simulink model "GunnerusDP_v1"  (R2017b)
settings: Solver=ode4  StartTime=0.0  StopTime=Tsim  FixedStep=ts  RelTol=1e-3  EnableMultiTasking=on
values from neighbouring files (symbols this model uses):
  ts = 0.01    [InitGunnerusDP.m]
undefined symbols (not defined in the file or in its folder): Control, Current, Hoerner, Par, Sim, TC_currentChange, vessel, vesselABC
libraries: marine_hydro x4, marine_gnc x3, simulink x3
(part 1 of 4)
settings Model: Creator=Thor  LastModifiedBy=astrbro
settings DataIOCC: LimitDataPoints=on  SaveFormat=Array  SignalLoggingSaveFormat=ModelDataLogs
settings OptimizationCC: ExpressionDepthLimit=2147483647  InitFltsAndDblsToZero=on  LifeSpan=inf
settings DebuggingCC: SaveWithParameterizedLinksMsg=none  UnderspecifiedInitializationDetection=Classic  MergeDetectMultiDrivingBlocksExec=none  SignalResolutionControl=TryResolveAllWithWarning  SolverPrmCheckMsg=warning  MultiTaskDSMMsg=warning  MultiTaskCondExecSysMsg=none  MultiTaskRateTransMsg=warning  FcnCallInpInsideContextMsg=warning  StateNameClashWarn=warning  SFUnexpectedBacktrackingDiag=warning  SFNoUnconditionalDefaultTransitionDiag=warning  SFExecutionAtInitializationDiag=none
settings HardwareCC: ProdBitPerPointer=32  ProdBitPerSizeT=32  ProdBitPerPtrDiffT=32  ProdLargestAtomicFloat=None  ProdIntDivRoundTo=Undefined  ProdEndianess=Unspecified  ProdWordSize=32  ProdHWDeviceType=32-bit Generic
settings ModelReferenceCC: PropagateSignalLabelsOutOfModel=off
settings CodeAppCC: StateflowObjectComments=on
settings GRTTargetCC: TargetFcnLib=ansi_tfl_tmw.mat  TargetLangStandard=C89/C90 (ANSI)  GeneratePreprocessorConditionals=Disable all  CombineOutputUpdateFcns=off  GRTInterface=on
settings ConfigComp: CovMetricSettings=dw  CovHtmlReporting=on  CovSaveCumulativeToWorkspaceVar=on  CovSaveSingleToWorkspaceVar=on  CovExternalEMLEnable=off  CovSFcnEnable=off

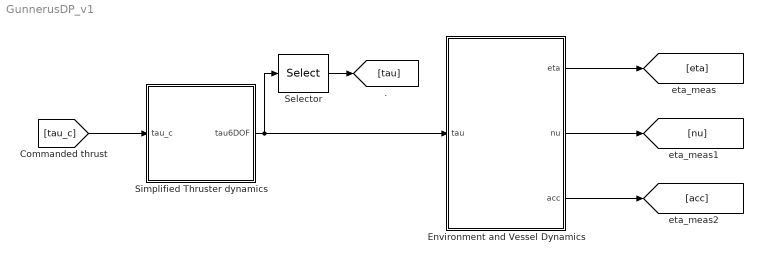
== system GunnerusDP_v1 ==
  Environment and Vessel Dynamics : Subsystem
  Selector : Selector  InputPortWidth=6  IndexOptions=Index vector (dialog)  Indices=[1 2 6]  OutputSizes=1
  Simplified Thruster dynamics : Subsystem
  wires:
  Selector/1 -> [tau]
  [tau_c] -> Simplified Thruster dynamics/1(tau_c)
  Simplified Thruster dynamics/1(tau6DOF) -> Selector/1, Environment and Vessel Dynamics/1(tau)
  Environment and Vessel Dynamics/2(nu) -> [nu]
  Environment and Vessel Dynamics/3(acc) -> [acc]
  Environment and Vessel Dynamics/1(eta) -> [eta]

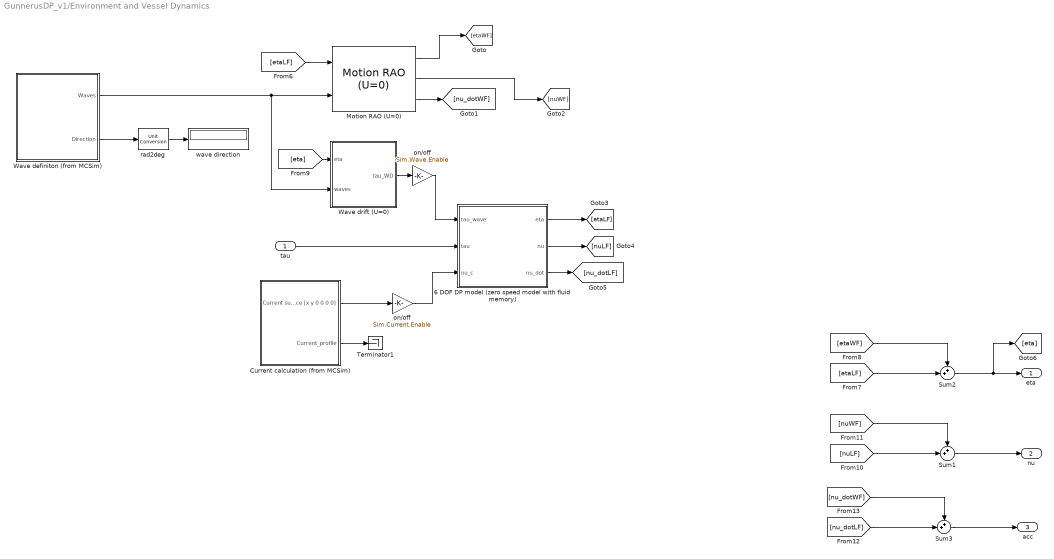
== system GunnerusDP_v1/Environment and Vessel Dynamics ==
  tau : Inport
  6 DOF DP model (zero speed model with fluid memory) : Subsystem  AncestorBlock=|  mask(6 DOF zero speed model){ABC=vesselABC, rho=1025, Axc=106, Ayc=419, CX=1.0, CY_2D=Hoerner(vessel.main.B,vessel.main.T), Bv=vessel.Bv, Dp=vesselABC.Dp}
      | marine_hydro/Hydro Library/6 DOF DP model
      |  (zero speed model with fluid memory)
      mask prompts: ABC "Structure containing model parameters and the fluid memory effects"; rho "Density of water (kg/m3)"; Axc "Frontal projected current area Axc (m2)"; Ayc "Laterall projected current area Ayc (m2)"; CX "Current (drag) coefficient in surge CX"; CY_2D "2D drag coefficient in sway CY_2D"; Bv "Linear viscous damping matrix"; Dp "Linear potential damping matrix"
      mask help: System block containing the zero speed 6 DOF equations of motion including fluid memory effetcs.
  Current calculation (from MCSim) : Subsystem
  Motion RAO (U=0) : marine_hydro/Hydro Library/Motion RAO (U=0)  RAO_Freq=vessel.motionRAO.w  RAO_Dir=vessel.headings  RAO_Vel=vessel.velocities  RAO_Amp=vessel.motionRAO.amp  RAO_Phase=vessel.motionRAO.phase  RAO_add_omega_0=on  RAO_add_omega_inf=on  RAO_yaw_quantization_flag=on  RAO_yaw_quant=5*pi/180  RAO_yaw_back=1.2*pi/180  RAO_speed_backlash_flag=on  RAO_speed_back=2  RAO_smoothing_flag=on
      settings: SourceProductName=MSS Hydro
  Sum1 : Sum  Inputs=++|
  Sum2 : Sum  Inputs=++|
  Sum3 : Sum  Inputs=++|
  Terminator1 : Terminator
  Wave definiton (from MCSim) : Subsystem
  Wave drift (U=0) : Subsystem  AncestorBlock=marine_hydro/Hydro Library/Wave drift (U=0)
  on/off : Gain  Gain=Sim.Wave.Enable
  "on/off " : Gain  Gain=Sim.Current.Enable
  rad2deg : marine_gnc/Utilities/Math Operations/Unit Conversion  in=rad2deg
      settings: SourceProductName=MSS GNC
  wave direction : Display
  eta : Outport
  nu : Outport  Port=2
  acc : Outport  Port=3
  wires:
  Current calculation (from MCSim)/2(Current_profile) -> Terminator1/1
  Wave drift (U=0)/1(tau_WD) -> on/off/1
  on/off/1 -> 6 DOF DP model (zero speed model with fluid memory)/1(tau_wave)
  "on/off "/1 -> 6 DOF DP model (zero speed model with fluid memory)/3(nu_c)
  Current calculation (from MCSim)/1(Current surface [x y 0 0 0 0]) -> "on/off "/1
  Motion RAO (U=0)/3 -> [nu_dotWF]
  Motion RAO (U=0)/2 -> [nuWF]
  Motion RAO (U=0)/1 -> [etaWF]
  rad2deg/1 -> wave direction/1
  Wave definiton (from MCSim)/2(Direction) -> rad2deg/1
  Wave definiton (from MCSim)/1(Waves) -> Motion RAO (U=0)/2, Wave drift (U=0)/2(waves)
  6 DOF DP model (zero speed model with fluid memory)/1(eta) -> [etaLF]
  tau/1 -> 6 DOF DP model (zero speed model with fluid memory)/2(tau)
  6 DOF DP model (zero speed model with fluid memory)/3(nu_dot) -> [nu_dotLF]
  6 DOF DP model (zero speed model with fluid memory)/2(nu) -> [nuLF]
  [etaLF] -> Motion RAO (U=0)/1
  [etaLF] -> Sum2/2
  [etaWF] -> Sum2/1
  Sum2/1 -> [eta], eta/1
  [eta] -> Wave drift (U=0)/1(eta)
  [nuLF] -> Sum1/2
  [nuWF] -> Sum1/1
  Sum1/1 -> nu/1
  [nu_dotLF] -> Sum3/2
  [nu_dotWF] -> Sum3/1
  Sum3/1 -> acc/1

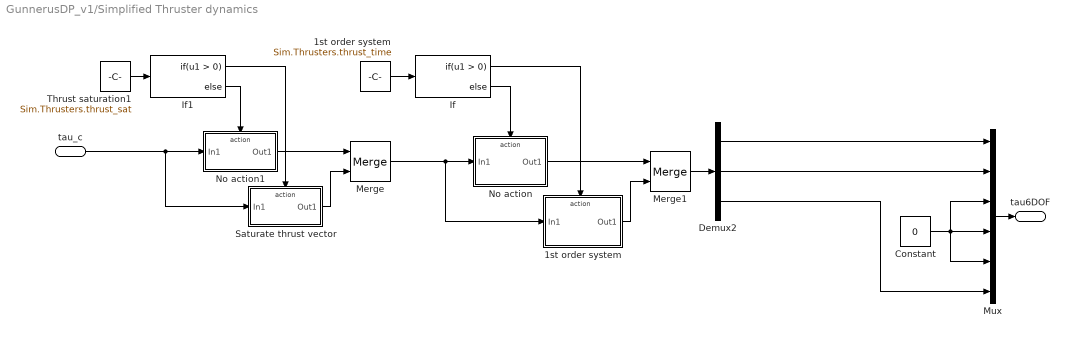
== system GunnerusDP_v1/Simplified Thruster dynamics ==
  tau_c : Inport
  "1st order system " : Constant  Value=Sim.Thrusters.thrust_time
  1st order system : Subsystem
  Constant : Constant  Value=0
  Demux2 : Demux  Outputs=3
  If : If
  If1 : If
  Merge : Merge
  Merge1 : Merge
  Mux : Mux  Inputs=6
  No action : Subsystem  TreatAsAtomicUnit=on
  No action1 : Subsystem  TreatAsAtomicUnit=on
  Saturate thrust vector : Subsystem  TreatAsAtomicUnit=on
  Thrust saturation1 : Constant  Value=Sim.Thrusters.thrust_sat
  tau6DOF : Outport  InitialOutput=[0,0,0,0,0,0]
  wires:
  Mux/1 -> tau6DOF/1
  Constant/1 -> Mux/3, Mux/4, Mux/5
  "1st order system "/1 -> If/1
  Thrust saturation1/1 -> If1/1
  No action1/1(Out1) -> Merge/1
  Saturate thrust vector/1(Out1) -> Merge/2
  If1/1 -> Saturate thrust vector/Action
  If1/2 -> No action1/Action
  Merge/1 -> 1st order system/1(In1), No action/1(In1)
  1st order system/1(Out1) -> Merge1/2
  No action/1(Out1) -> Merge1/1
  If/2 -> No action/Action
  If/1 -> 1st order system/Action
  Merge1/1 -> Demux2/1
  Demux2/1 -> Mux/1
  Demux2/2 -> Mux/2
  Demux2/3 -> Mux/6
  tau_c/1 -> Saturate thrust vector/1(In1), No action1/1(In1)

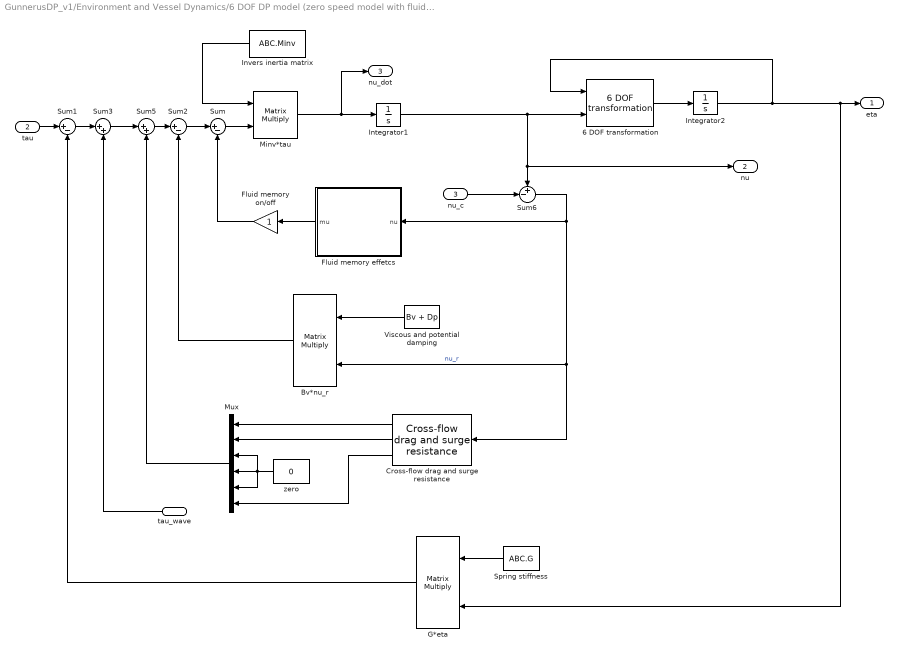
== system GunnerusDP_v1/Environment and Vessel Dynamics/6 DOF DP model (zero speed model with fluid memory) ==
  tau_wave : Inport
  tau : Inport  Port=2
  nu_c : Inport  Port=3
  6 DOF transformation : marine_gnc/Models/ Kinematics/6 DOF transformation
      settings: SourceProductName=MSS GNC
  Bv*nu_r : Product  Multiplication=Matrix(*)  SaturateOnIntegerOverflow=on  OutDataTypeStr=Inherit: Same as first input
  Cross-flow drag and surge resistance : marine_hydro/Hydro Library/Cross-flow drag and surge resistance  N=20  Lpp=vessel.main.Lpp  CD=CY_2D  Cx=CX  Ax=Axc  Ay=Ayc  rho_w=rho
      settings: SourceProductName=MSS Hydro
  Fluid memory effetcs : Subsystem
  Fluid memory on/off : Gain
  G*eta : Product  Multiplication=Matrix(*)  SaturateOnIntegerOverflow=on  OutDataTypeStr=Inherit: Same as first input
  "Integrator1 " : Integrator
  Integrator2 : Integrator
  Invers inertia matrix : Constant  Value=ABC.Minv
  Minv*tau : Product  Inputs=**  Multiplication=Matrix(*)  SaturateOnIntegerOverflow=on  OutDataTypeStr=Inherit: Same as first input
  Mux : Mux  Inputs=6
  Spring stiffness : Constant  Value=ABC.G
  Sum : Sum  Inputs=|+-  SaturateOnIntegerOverflow=on
  Sum1 : Sum  Inputs=|+-  SaturateOnIntegerOverflow=on
  Sum2 : Sum  Inputs=|+-  SaturateOnIntegerOverflow=on
  Sum3 : Sum  Inputs=|++  SaturateOnIntegerOverflow=on
  Sum5 : Sum  Inputs=|++  SaturateOnIntegerOverflow=on
  Sum6 : Sum  Inputs=+-|  SaturateOnIntegerOverflow=on
  Viscous and potential damping : Constant  Value=Bv + Dp
  zero : Constant  Value=0
  eta : Outport
  nu : Outport  Port=2
  nu_dot : Outport  Port=3
  wires:
  Sum5/1 -> Sum2/1
  Fluid memory effetcs/1(mu) -> Fluid memory on/off/1
  Sum3/1 -> Sum5/1
  tau_wave/1 -> Sum3/2
  tau/1 -> Sum1/1
  G*eta/1 -> Sum1/2
  Integrator2/1 -> 6 DOF transformation/1, G*eta/2, eta/1
  6 DOF transformation/1 -> Integrator2/1
  Minv*tau/1 -> nu_dot/1, "Integrator1 "/1
  Invers inertia matrix/1 -> Minv*tau/1
  Spring stiffness/1 -> G*eta/1
  Sum1/1 -> Sum3/1
  Sum/1 -> Minv*tau/2
  "Integrator1 "/1 -> 6 DOF transformation/2, nu/1, Sum6/1
  Cross-flow drag and surge resistance/1 -> Mux/1
  Cross-flow drag and surge resistance/2 -> Mux/2
  Cross-flow drag and surge resistance/3 -> Mux/6
  zero/1 -> Mux/4, Mux/3, Mux/5
  Mux/1 -> Sum5/2
  nu_c/1 -> Sum6/2
  Sum6/1 -> Fluid memory effetcs/1(nu), Cross-flow drag and surge resistance/1, Bv*nu_r/2  "nu_r"
  Viscous and potential damping/1 -> Bv*nu_r/1
  Sum2/1 -> Sum/1
  Bv*nu_r/1 -> Sum2/2
  Fluid memory on/off/1 -> Sum/2

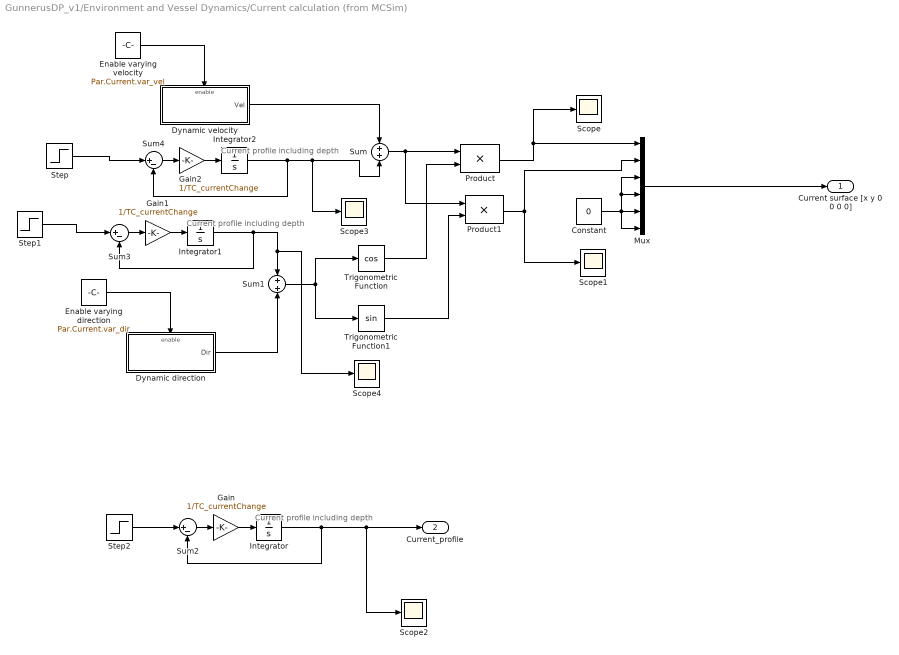
== system GunnerusDP_v1/Environment and Vessel Dynamics/Current calculation (from MCSim) ==
  note: Current profile including depth
  note: Current profile including depth
  note: Current profile including depth
  Constant : Constant  Value=0
  Dynamic direction : Subsystem  TreatAsAtomicUnit=on
  Dynamic velocity : Subsystem  TreatAsAtomicUnit=on
  Enable varying direction : Constant  Value=Par.Current.var_dir  VectorParams1D=off
  Enable varying velocity : Constant  Value=Par.Current.var_vel  VectorParams1D=off
  Gain : Gain  Gain=1/TC_currentChange
  Gain1 : Gain  Gain=1/TC_currentChange
  Gain2 : Gain  Gain=1/TC_currentChange
  Integrator : Integrator
  Integrator1 : Integrator
  Integrator2 : Integrator
  Mux : Mux  Inputs=6
  Product : Product  SaturateOnIntegerOverflow=on  OutDataTypeStr=Inherit: Same as first input
  Product1 : Product  SaturateOnIntegerOverflow=on  OutDataTypeStr=Inherit: Same as first input
  Scope{,1..4} (5 alike) : Scope
  Step : Step  Time=Current.Change.Time  Before=Par.Current.vel  After=Par.Current.vel2  SampleTime=ts
  Step1 : Step  Time=Current.Change.Time  Before=Par.Current.dir  After=Par.Current.dir2  SampleTime=ts
  Step2 : Step  Time=Current.Change.Time  Before=Par.Current.Profile  After=Par.Current.Profile2  SampleTime=ts
  Sum : Sum  SaturateOnIntegerOverflow=on
  Sum1 : Sum  SaturateOnIntegerOverflow=on
  Sum2 : Sum  Inputs=|+-
  Sum3 : Sum  Inputs=|+-
  Sum4 : Sum  Inputs=|+-
  Trigonometric Function : Trigonometry  Operator=cos
  Trigonometric Function1 : Trigonometry
  Current surface [x y 0 0 0 0] : Outport
  Current_profile : Outport  Port=2
  wires:
  Enable varying velocity/1 -> Dynamic velocity/Enable
  Sum1/1 -> Trigonometric Function/1, Trigonometric Function1/1
  Product/1 -> Mux/1, Scope/1
  Product1/1 -> Mux/2, Scope1/1
  Sum/1 -> Product/1, Product1/1
  Trigonometric Function/1 -> Product/2
  Trigonometric Function1/1 -> Product1/2
  Mux/1 -> Current surface [x y 0 0 0 0]/1
  Enable varying direction/1 -> Dynamic direction/Enable
  Dynamic direction/1(Dir) -> Sum1/2
  Dynamic velocity/1(Vel) -> Sum/1
  Integrator/1 -> Sum2/2, Scope2/1, Current_profile/1
  Step2/1 -> Sum2/1
  Sum2/1 -> Gain/1
  Gain/1 -> Integrator/1
  Integrator1/1 -> Scope4/1, Sum1/1, Sum3/2
  Step1/1 -> Sum3/1
  Sum3/1 -> Gain1/1
  Gain1/1 -> Integrator1/1
  Integrator2/1 -> Sum4/2, Scope3/1, Sum/2
  Step/1 -> Sum4/1
  Sum4/1 -> Gain2/1
  Gain2/1 -> Integrator2/1
  Constant/1 -> Mux/6, Mux/5, Mux/4, Mux/3

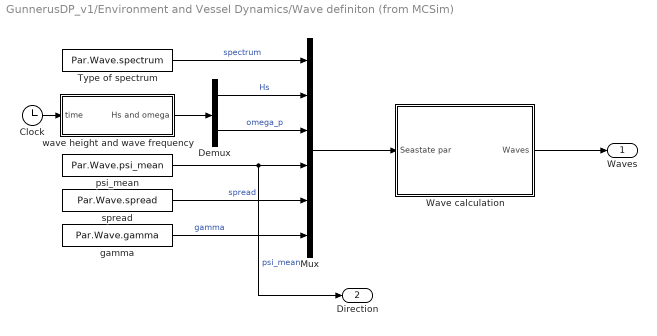
== system GunnerusDP_v1/Environment and Vessel Dynamics/Wave definiton (from MCSim) ==
  Clock : Clock
  Demux : Demux  Outputs=2
  Mux : Mux  Inputs=6
  Type of spectrum : Constant  Value=Par.Wave.spectrum
  Wave calculation : Subsystem  mask(Wave calculation){nwaves=Par.Wave.nwave, nfreq=Par.Wave.nfreq, ndir=Par.Wave.ndir, randfreq_flag=Par.Wave.rand_freq, randdir_flag=Par.Wave.rand_dir, rand_seed=133, freq_cutoff=Par.Wave.cutoff, dir_cutoff=Par.Wave.cutoff_dir}
      mask prompts: nwaves "Number of waves (<=nfreq*ndir)"; nfreq "Number of frequencies in grid (recommended > 20)"; ndir "Number of directions in grid (>= 1)"; randfreq_flag "Random frequency flag {0,1}"; randdir_flag "Random direction flag {0,1}"; rand_seed "Random number seed (integer)"; freq_cutoff "Frequency cutoff factor [1.5, 5], default 3"; dir_cutoff "Direction cutoff [0, 3pi/8], default 0"
      mask help:
      | Calculate wave components from input sea state parameters:
      |
      | Seastate par(1):	Spectrum type {1,2,3}
      | Seastate par(2):	Significant wave height [m] [0, 15]
      | Seastate par(3):	Peak frequency [rad/s]
      | Seastate par(4):	Mean wave direction [rad]
      | Seastate par(5):	Wave spreading factor {1,2,3,4,5}
      | Seastate par(6):	Gamma [1, 7] (default 3.3)
      |
      | The frequency spectrum types are:
      |
      | -1- Modified Pierson Moskowitz (ITTC/ISSC)
      | -2- JONSWAP
      | -3- Torsethaugen doubly peaked
      |
      | Input spreading factor 0 and one wave direction in the mask to get long-crested waves (all wave energy in one direction).
      |
      | Input negative or zero peak frequency to get an expectation value from the significant wave height, based on north sea statistical data.
      |
      | The spectrum type, spreading factor or gamma should not be changed online unless the significant wave heigth is zero.
      |
      | Author: Øyvind Notland Smogeli, 2004
      |
      | Copyright Marine Cybernetics AS 2004
      mask Help:
      | <p>Calculate wave components from input sea state parameters:<br>
      | <br>
      | Seastate par(1):&nbsp;&nbsp;&nbsp;&nbsp; Spectrum type {1,2,3}<br>
      | Seastate par(2):&nbsp;&nbsp;&nbsp;&nbsp; Significant wave height [m] [0, 15]<br>
      | Seastate par(3):&nbsp;&nbsp;&nbsp;&nbsp; Peak frequency [rad/s]<br>
      | Seastate par(4):&nbsp;&nbsp;&nbsp;&nbsp; Mean wave direction [rad]<br>
      | Seastate par(5):&nbsp;&nbsp;&nbsp;&nbsp; Wave spreading factor {1,2,3,4,5} <br>
      | Seastate par(6):&nbsp;&nbsp;&nbsp;&nbsp; Gamma [1, 7] (default 3.3)<br>
      | <br>
      | The directional spectrum centers the wave energy around the mean<br>
      | direction for large spreading factor, and spreads the energy out<br>
      | for low spreading factors. 1 is recommended by ITTC, 2 by ISSC.<br>
      | <br>
      | The freqeuncy cutoff factor sets the max frequency in the spectrum<br>
      | as: omega_max = cutoff*omega_peak.<br>
      | 4 is recommended for the Torsethaugen spectrum, 3 for the others.<br>
      | <br>
      | The direction cutoff skips the outer directions in the direction<br>
      | spectrum, such that the span [-(pi/2-dir_cutoff) (pi/2-dir_cutoff)]<br>
      | is used around the mean direction. The direction cutoff should be<br>
      | set in correspondence with the minimum spreading factor to<br>
      | be used in the simulation (with a large spreading factor the<br>
      | direction cutoff may be increased without removing any<br>
      | significant waves).<br>
      | <br>
      | With correctly tuned frequency and direction cutoff, the number<br>
      | of directions and frequencies in the grid may be decreased<br>
      | without affecting the resolution of the grid.<br>
      | <br>
      | The peakness factor is valid in the range [0,1]. For 1, the JONSWAP<br>
      | spectrum is equal to the PM spectrum, and for inceasing peakness<br>
      | factor the spectrum becomes more peaked.<br>
      | <br>
      | Input spreading factor 0 and one wave direction in the mask to get<br>
      | long-crested waves (all wave energy in one direction).<br>
      | <br>
      | Input negative or zero peak frequency to get an expectation value<br>
      | from the significant wave height, based on north sea statistical data.<br>
      | <br>
      | The spectrum type should not be changed online unless the <br>
      | significant wave heigth is zero.</p>
      | <br>
      | The executable wave_calculation.dll must be on your matlab path.<br>
      | <br>
      | Author: Øyvind Notland Smogeli, 2004<br>
      | <br>
      | Copyright Marine Cybernetics AS 2004<br>
  gamma : Constant  Value=Par.Wave.gamma
  psi_mean : Constant  Value=Par.Wave.psi_mean
  spread : Constant  Value=Par.Wave.spread
  wave height and wave frequency : Subsystem
  Waves : Outport
  Direction : Outport  Port=2
  wires:
  Wave calculation/1(Waves) -> Waves/1
  psi_mean/1 -> Direction/1, Mux/4  "psi_mean"
  spread/1 -> Mux/5  "spread"
  gamma/1 -> Mux/6  "gamma"
  Type of spectrum/1 -> Mux/1  "spectrum"
  Mux/1 -> Wave calculation/1(Seastate par)
  Clock/1 -> wave height and wave frequency/1(time)
  Demux/1 -> Mux/2  "Hs"
  Demux/2 -> Mux/3  "omega_p"
  wave height and wave frequency/1(Hs and omega) -> Demux/1

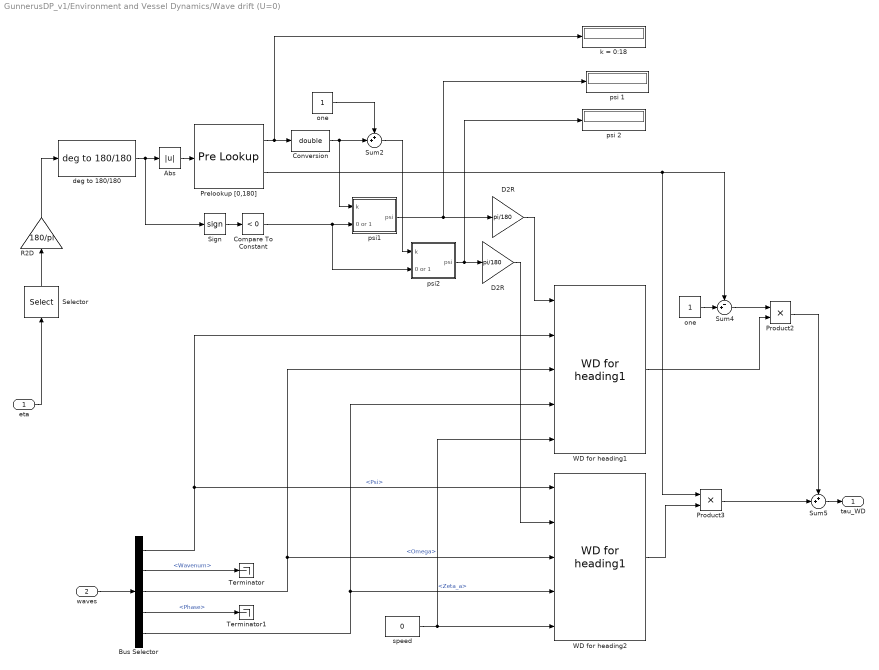
== system GunnerusDP_v1/Environment and Vessel Dynamics/Wave drift (U=0) ==
  eta : Inport
  waves : Inport  Port=2
  Abs : Abs  SaturateOnIntegerOverflow=on
  Bus Selector : BusSelector  OutputSignals=Psi,Wavenum,Omega,Phase,Zeta_a
  Compare To Constant : simulink/Logic and Bit Operations/Compare To Constant  relop=<  const=0  OutDataTypeStr=uint8  ZeroCross=off
  Conversion : DataTypeConversion  OutDataTypeStr=double
  D2R : Gain  Gain=pi/180
  "D2R " : Gain  Gain=pi/180
  Prelookup [0,180] : PreLookup  BreakpointsData=[0:10:180]  IndexSearchMethod=Evenly spaced points  BeginIndexSearchUsingPreviousIndexResult=on
  Product2 : Product  RndMeth=Zero
  Product3 : Product  RndMeth=Zero
  R2D : Gain  Gain=180/pi
  Selector : Selector  InputPortWidth=6  IndexOptions=Index vector (dialog)  Indices=[6]  OutputSizes=1
  Sign : Signum
  Sum2 : Sum  Inputs=++|
  Sum4 : Sum  Inputs=-+|
  Sum5 : Sum  Inputs=++|
  Terminator : Terminator
  Terminator1 : Terminator
  WD for heading1 : marine_hydro/Hydro Library/WD for heading1  ForceRAO_Freq=vessel.forceRAO.w  WD_Freq=vessel.driftfrc.w  RAO_Vel=vessel.velocities  ForceRAO_Amp=vessel.forceRAO.amp  ForceRAO_Phase=vessel.forceRAO.phase  WD_Amp=vessel.driftfrc.amp  RAO_add_omega_0=on  RAO_add_omega_inf=on
      settings: SourceProductName=MSS Hydro
  WD for heading2 : marine_hydro/Hydro Library/WD for heading1  ForceRAO_Freq=vessel.forceRAO.w  WD_Freq=vessel.driftfrc.w  RAO_Vel=vessel.velocities  ForceRAO_Amp=vessel.forceRAO.amp  ForceRAO_Phase=vessel.forceRAO.phase  WD_Amp=vessel.driftfrc.amp  RAO_add_omega_0=on  RAO_add_omega_inf=on
      settings: SourceProductName=MSS Hydro
  deg to 180/180 : marine_gnc/Utilities/Math Operations/deg to 180//180
      settings: SourceProductName=MSS GNC
  k = 0:18 : Display
  one : Constant
  "one " : Constant
  psi 1 : Display
  psi 2 : Display
  psi1 : Subsystem
  psi2 : Subsystem
  speed : Constant  Value=0
  tau_WD : Outport
  wires:
  WD for heading2/1 -> Product3/2
  eta/1 -> Selector/1
  "one "/1 -> Sum4/2
  Sum4/1 -> Product2/1
  WD for heading1/1 -> Product2/2
  Product3/1 -> Sum5/2
  Product2/1 -> Sum5/1
  Prelookup [0,180]/1 -> Conversion/1, k = 0:18/1
  one/1 -> Sum2/1
  Sum2/1 -> psi2/1(k)
  deg to 180/180/1 -> Abs/1, Sign/1
  Abs/1 -> Prelookup [0,180]/1
  Sign/1 -> Compare To Constant/1
  Compare To Constant/1 -> psi1/2(0 or 1), psi2/2(0 or 1)
  psi1/1(psi) -> D2R/1, psi 1/1
  Prelookup [0,180]/2 -> Product3/1, Sum4/1
  Conversion/1 -> Sum2/2, psi1/1(k)
  psi2/1(psi) -> "D2R "/1, psi 2/1
  waves/1 -> Bus Selector/1
  Sum5/1 -> tau_WD/1
  Selector/1 -> R2D/1
  R2D/1 -> deg to 180/180/1
  speed/1 -> WD for heading2/5, WD for heading1/5
  Bus Selector/3 -> WD for heading2/3, WD for heading1/3  "<Omega>"
  Bus Selector/5 -> WD for heading2/4, WD for heading1/4  "<Zeta_a>"
  Bus Selector/2 -> Terminator/1  "<Wavenum>"
  Bus Selector/1 -> WD for heading1/2, WD for heading2/1  "<Psi>"
  Bus Selector/4 -> Terminator1/1  "<Phase>"
  D2R/1 -> WD for heading1/1
  "D2R "/1 -> WD for heading2/2

== system GunnerusDP_v1/Simplified Thruster dynamics/1st order system ==
  In1 : Inport
  Action Port : ActionPort  ActionType=then
  1st order system : TransferFcn  Denominator=[Sim.Thrusters.T_surge 1]
  1st order system1 : TransferFcn  Denominator=[Sim.Thrusters.T_sway 1]
  1st order system2 : TransferFcn  Denominator=[Sim.Thrusters.T_yaw 1]
  Demux : Demux  Outputs=3
  Mux4 : Mux  Inputs=3
  Out1 : Outport
  wires:
  Demux/1 -> 1st order system/1
  Demux/2 -> 1st order system1/1
  Demux/3 -> 1st order system2/1
  1st order system/1 -> Mux4/1
  1st order system1/1 -> Mux4/2
  1st order system2/1 -> Mux4/3
  In1/1 -> Demux/1
  Mux4/1 -> Out1/1

== system GunnerusDP_v1/Simplified Thruster dynamics/No action ==
  In1 : Inport
  Action Port : ActionPort  ActionType=else
  Out1 : Outport
  wires:
  In1/1 -> Out1/1

== system GunnerusDP_v1/Simplified Thruster dynamics/No action1 ==
  In1 : Inport
  Action Port : ActionPort  ActionType=else
  Out1 : Outport
  wires:
  In1/1 -> Out1/1

== system GunnerusDP_v1/Simplified Thruster dynamics/Saturate thrust vector ==
  In1 : Inport
  Action Port : ActionPort  ActionType=then
  Saturation : Saturate  UpperLimit=Control.Tau_max  LowerLimit=-Control.Tau_max
  Out1 : Outport
  wires:
  In1/1 -> Saturation/1
  Saturation/1 -> Out1/1

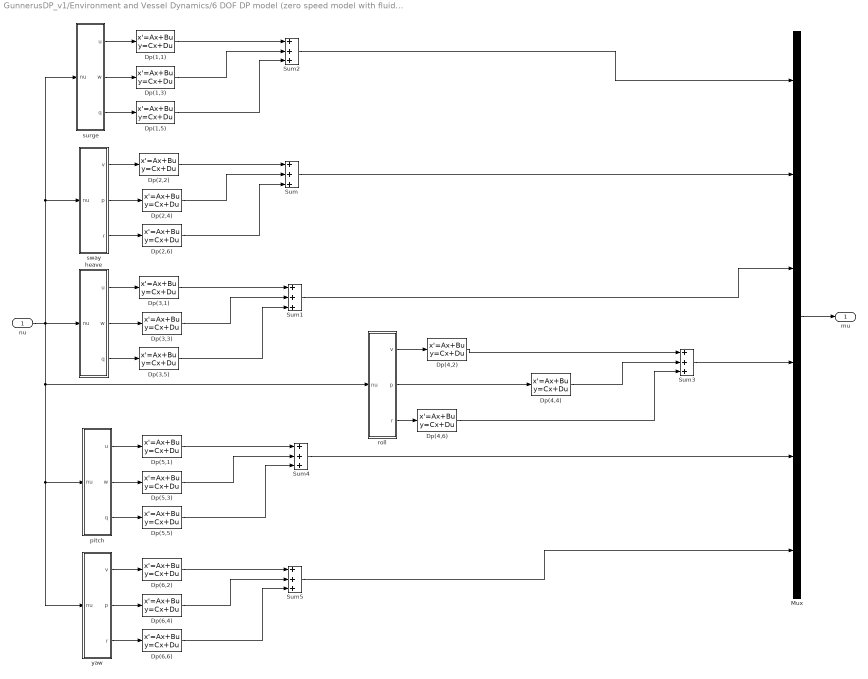
== system GunnerusDP_v1/Environment and Vessel Dynamics/6 DOF DP model (zero speed model with fluid memory)/Fluid memory effetcs ==
  nu : Inport
  Dp(1,1) : StateSpace  A=ABC.Ar{1,1}  B=ABC.Br{1,1}  C=ABC.Cr{1,1}  D=ABC.Dr{1,1}  InitialCondition=0
  Dp(1,3) : StateSpace  A=ABC.Ar{1,3}  B=ABC.Br{1,3}  C=ABC.Cr{1,3}  D=ABC.Dr{1,3}  InitialCondition=0
  Dp(1,5) : StateSpace  A=ABC.Ar{1,5}  B=ABC.Br{1,5}  C=ABC.Cr{1,5}  D=ABC.Dr{1,5}  InitialCondition=0
  Dp(2,2) : StateSpace  A=ABC.Ar{2,2}  B=ABC.Br{2,2}  C=ABC.Cr{2,2}  D=ABC.Dr{2,2}  InitialCondition=0
  Dp(2,4) : StateSpace  A=ABC.Ar{2,4}  B=ABC.Br{2,4}  C=ABC.Cr{2,4}  D=ABC.Dr{2,4}  InitialCondition=0
  Dp(2,6) : StateSpace  A=ABC.Ar{2,6}  B=ABC.Br{2,6}  C=ABC.Cr{2,6}  D=ABC.Dr{2,6}  InitialCondition=0
  Dp(3,1) : StateSpace  A=ABC.Ar{3,1}  B=ABC.Br{3,1}  C=ABC.Cr{3,1}  D=ABC.Dr{3,1}  InitialCondition=0
  Dp(3,3) : StateSpace  A=ABC.Ar{3,3}  B=ABC.Br{3,3}  C=ABC.Cr{3,3}  D=ABC.Dr{3,3}  InitialCondition=0
  Dp(3,5) : StateSpace  A=ABC.Ar{3,5}  B=ABC.Br{3,5}  C=ABC.Cr{3,5}  D=ABC.Dr{3,5}  InitialCondition=0
  Dp(4,2) : StateSpace  A=ABC.Ar{4,2}  B=ABC.Br{4,2}  C=ABC.Cr{4,2}  D=ABC.Dr{4,2}  InitialCondition=0
  Dp(4,4) : StateSpace  A=ABC.Ar{4,4}  B=ABC.Br{4,4}  C=ABC.Cr{4,4}  D=ABC.Dr{4,4}  InitialCondition=0
  Dp(4,6) : StateSpace  A=ABC.Ar{4,6}  B=ABC.Br{4,6}  C=ABC.Cr{4,6}  D=ABC.Dr{4,6}  InitialCondition=0
  Dp(5,1) : StateSpace  A=ABC.Ar{5,1}  B=ABC.Br{5,1}  C=ABC.Cr{5,1}  D=ABC.Dr{5,1}  InitialCondition=0
  Dp(5,3) : StateSpace  A=ABC.Ar{5,3}  B=ABC.Br{5,3}  C=ABC.Cr{5,3}  D=ABC.Dr{5,3}  InitialCondition=0
  Dp(5,5) : StateSpace  A=ABC.Ar{5,5}  B=ABC.Br{5,5}  C=ABC.Cr{5,5}  D=ABC.Dr{5,5}  InitialCondition=0
  Dp(6,2) : StateSpace  A=ABC.Ar{6,2}  B=ABC.Br{6,2}  C=ABC.Cr{6,2}  D=ABC.Dr{6,2}  InitialCondition=0
  Dp(6,4) : StateSpace  A=ABC.Ar{6,4}  B=ABC.Br{6,4}  C=ABC.Cr{6,4}  D=ABC.Dr{6,4}  InitialCondition=0
  Dp(6,6) : StateSpace  A=ABC.Ar{6,6}  B=ABC.Br{6,6}  C=ABC.Cr{6,6}  D=ABC.Dr{6,6}  InitialCondition=0
  Mux : Mux  Inputs=6
  Sum{,1..5} (6 alike) : Sum  Inputs=+++  SaturateOnIntegerOverflow=on
  heave : Subsystem
  pitch : Subsystem
  roll : Subsystem
  surge : Subsystem
  sway : Subsystem
  yaw : Subsystem
  mu : Outport
  wires:
  Dp(4,4)/1 -> Sum3/2
  roll/2(p) -> Dp(4,4)/1
  Sum5/1 -> Mux/6
  yaw/3(r) -> Dp(6,6)/1
  yaw/2(p) -> Dp(6,4)/1
  yaw/1(v) -> Dp(6,2)/1
  Dp(6,6)/1 -> Sum5/3
  Dp(6,4)/1 -> Sum5/2
  Dp(6,2)/1 -> Sum5/1
  Sum3/1 -> Mux/4
  Dp(5,1)/1 -> Sum4/1
  pitch/1(u) -> Dp(5,1)/1
  pitch/2(w) -> Dp(5,3)/1
  pitch/3(q) -> Dp(5,5)/1
  Dp(5,5)/1 -> Sum4/3
  Dp(5,3)/1 -> Sum4/2
  roll/3(r) -> Dp(4,6)/1
  roll/1(v) -> Dp(4,2)/1
  Dp(4,6)/1 -> Sum3/3
  Dp(4,2)/1 -> Sum3/1
  Dp(1,1)/1 -> Sum2/1
  surge/1(u) -> Dp(1,1)/1
  surge/2(w) -> Dp(1,3)/1
  surge/3(q) -> Dp(1,5)/1
  Sum2/1 -> Mux/1
  Dp(1,5)/1 -> Sum2/3
  Dp(1,3)/1 -> Sum2/2
  Mux/1 -> mu/1
  nu/1 -> yaw/1(nu), pitch/1(nu), roll/1(nu), surge/1(nu), sway/1(nu), heave/1(nu)
  Dp(3,1)/1 -> Sum1/1
  heave/1(u) -> Dp(3,1)/1
  heave/2(w) -> Dp(3,3)/1
  heave/3(q) -> Dp(3,5)/1
  Sum1/1 -> Mux/3
  Dp(3,5)/1 -> Sum1/3
  Dp(3,3)/1 -> Sum1/2
  sway/3(r) -> Dp(2,6)/1
  sway/2(p) -> Dp(2,4)/1
  sway/1(v) -> Dp(2,2)/1
  Sum/1 -> Mux/2
  Dp(2,6)/1 -> Sum/3
  Dp(2,4)/1 -> Sum/2
  Dp(2,2)/1 -> Sum/1
  Sum4/1 -> Mux/5

== system GunnerusDP_v1/Environment and Vessel Dynamics/Current calculation (from MCSim)/Dynamic direction ==
  Enable : EnablePort
  Band-Limited White Noise : simulink/Sources/Band-Limited White Noise  Cov=Par.Current.wn_p_dir  Ts=Par.Current.wn_t_dir  seed=Par.Current.wn_s_dir
  Integrator : Integrator  LimitOutput=on  UpperSaturationLimit=Par.Current.sat_dir  LowerSaturationLimit=-Par.Current.sat_dir
  Sum : Sum  Inputs=|+-  SaturateOnIntegerOverflow=on
  mju_dir : Gain  Gain=Par.Current.mju_dir  SampleTime=ts  SaturateOnIntegerOverflow=on  OutDataTypeStr=Inherit: Same as input  ParamDataTypeStr=Inherit: Same as input
  Dir : Outport  InitialOutput=0
  wires:
  Band-Limited White Noise/1 -> Sum/1  "w"
  Sum/1 -> Integrator/1  "psi_dot"
  Integrator/1 -> Dir/1, mju_dir/1  "psi"
  mju_dir/1 -> Sum/2

== system GunnerusDP_v1/Environment and Vessel Dynamics/Current calculation (from MCSim)/Dynamic velocity ==
  Enable : EnablePort
  Band-Limited White Noise : simulink/Sources/Band-Limited White Noise  Cov=Par.Current.wn_p_vel  Ts=Par.Current.wn_t_vel  seed=Par.Current.wn_s_vel
  Integrator : Integrator  LimitOutput=on  UpperSaturationLimit=Par.Current.sat_vel  LowerSaturationLimit=-Par.Current.sat_vel
  Sum : Sum  Inputs=|+-  SaturateOnIntegerOverflow=on
  mju_vel : Gain  Gain=Par.Current.mju_vel  SampleTime=ts  SaturateOnIntegerOverflow=on  OutDataTypeStr=Inherit: Same as input  ParamDataTypeStr=Inherit: Same as input
  Vel : Outport  InitialOutput=0
  wires:
  Band-Limited White Noise/1 -> Sum/1  "w"
  Sum/1 -> Integrator/1  "v_dot"
  Integrator/1 -> mju_vel/1, Vel/1  "v"
  mju_vel/1 -> Sum/2

== system GunnerusDP_v1/Environment and Vessel Dynamics/Wave definiton (from MCSim)/Wave calculation ==
  Seastate par : Inport
  Bus Creator : BusCreator  Inputs=5
  S-Function : S-Function  FunctionName=wave_calculation  Parameters=[nwaves, nfreq, ndir, randfreq_flag, randdir_flag, rand_seed, freq_cutoff, dir_cutoff]  SFunctionDeploymentMode=off  EnableBusSupport=off  mask(Wave_calculation s-function mask){nwaves=nwaves, nfreq=nfreq, ndir=ndir, randfreq_flag=randfreq_flag, randdir_flag=randdir_flag, rand_seed=rand_seed, freq_cutoff=freq_cutoff, dir_cutoff=dir_cutoff}
      mask prompts: nwaves "Number of waves (<=nfreq*ndir)"; nfreq "Number of frequencies in grid (recommended > 20)"; ndir "Number of directions in grid (>= 1)"; randfreq_flag "Random frequency flag {0,1}"; randdir_flag "Random direction flag {0,1}"; rand_seed "Random number seed (integer)"; freq_cutoff "Frequency cutoff factor [1.5, 5], default 3"; dir_cutoff "Direction cutoff [0, 3pi/8], default 0"
      mask Display:
      | port_label('input', 1, 'Seastate par')
      | port_label('output', 1, 'Omega')
      | port_label('output', 2, 'Psi')
      | port_label('output', 3, 'Zeta_a')
      | port_label('output', 4, 'Wavenum')
      | port_label('output', 5, 'Phase')
  Scope : Scope
  Scope1 : Scope
  Waves : Outport
  wires:
  Seastate par/1 -> S-Function/1
  Bus Creator/1 -> Waves/1
  S-Function/4 -> Bus Creator/4  "Wavenum"
  S-Function/3 -> Bus Creator/3, Scope1/1  "Zeta_a"
  S-Function/2 -> Bus Creator/2  "Psi"
  S-Function/1 -> Bus Creator/1, Scope/1  "Omega"
  S-Function/5 -> Bus Creator/5  "Phase"

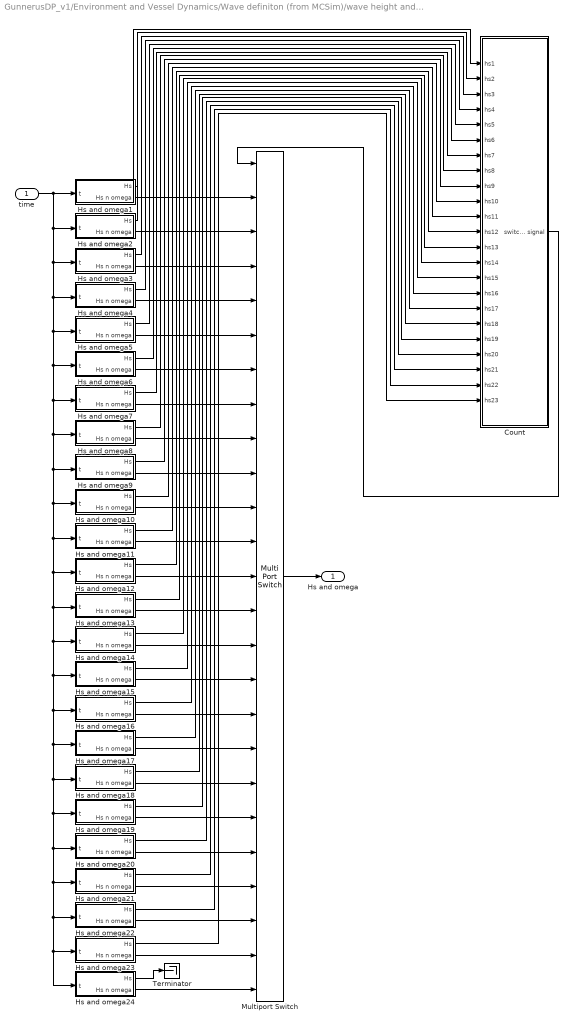
== system GunnerusDP_v1/Environment and Vessel Dynamics/Wave definiton (from MCSim)/wave height and wave frequency ==
  time : Inport
  Count : Subsystem
  Hs and omega1 : Subsystem
  Hs and omega10 : Subsystem
  Hs and omega11 : Subsystem
  Hs and omega12 : Subsystem
  Hs and omega13 : Subsystem
  Hs and omega14 : Subsystem
  Hs and omega15 : Subsystem
  Hs and omega16 : Subsystem
  Hs and omega17 : Subsystem
  Hs and omega18 : Subsystem
  Hs and omega19 : Subsystem
  Hs and omega2 : Subsystem
  Hs and omega20 : Subsystem
  Hs and omega21 : Subsystem
  Hs and omega22 : Subsystem
  Hs and omega23 : Subsystem
  Hs and omega24 : Subsystem
  Hs and omega3 : Subsystem
  Hs and omega4 : Subsystem
  Hs and omega5 : Subsystem
  Hs and omega6 : Subsystem
  Hs and omega7 : Subsystem
  Hs and omega8 : Subsystem
  Hs and omega9 : Subsystem
  Multiport Switch : MultiPortSwitch  Inputs=24  SaturateOnIntegerOverflow=on
  Terminator : Terminator
  Hs and omega : Outport
  wires:
  time/1 -> Hs and omega2/1(t), Hs and omega3/1(t), Hs and omega4/1(t), Hs and omega5/1(t), Hs and omega6/1(t), Hs and omega7/1(t), Hs and omega8/1(t), Hs and omega9/1(t), Hs and omega10/1(t), Hs and omega11/1(t), Hs and omega12/1(t), Hs and omega13/1(t), Hs and omega14/1(t), Hs and omega15/1(t), Hs and omega16/1(t), Hs and omega17/1(t), Hs and omega18/1(t), Hs and omega19/1(t), Hs and omega20/1(t), Hs and omega21/1(t), Hs and omega22/1(t), Hs and omega24/1(t), Hs and omega23/1(t), Hs and omega1/1(t)
  Hs and omega1/2(Hs n omega) -> Multiport Switch/2
  Hs and omega2/2(Hs n omega) -> Multiport Switch/3
  Hs and omega3/2(Hs n omega) -> Multiport Switch/4
  Hs and omega4/2(Hs n omega) -> Multiport Switch/5
  Hs and omega5/2(Hs n omega) -> Multiport Switch/6
  Hs and omega6/2(Hs n omega) -> Multiport Switch/7
  Hs and omega7/2(Hs n omega) -> Multiport Switch/8
  Hs and omega8/2(Hs n omega) -> Multiport Switch/9
  Hs and omega9/2(Hs n omega) -> Multiport Switch/10
  Hs and omega10/2(Hs n omega) -> Multiport Switch/11
  Hs and omega11/2(Hs n omega) -> Multiport Switch/12
  Hs and omega12/2(Hs n omega) -> Multiport Switch/13
  Hs and omega13/2(Hs n omega) -> Multiport Switch/14
  Hs and omega14/2(Hs n omega) -> Multiport Switch/15
  Hs and omega15/2(Hs n omega) -> Multiport Switch/16
  Hs and omega16/2(Hs n omega) -> Multiport Switch/17
  Hs and omega17/2(Hs n omega) -> Multiport Switch/18
  Hs and omega18/2(Hs n omega) -> Multiport Switch/19
  Hs and omega19/2(Hs n omega) -> Multiport Switch/20
  Hs and omega20/2(Hs n omega) -> Multiport Switch/21
  Hs and omega21/2(Hs n omega) -> Multiport Switch/22
  Hs and omega22/2(Hs n omega) -> Multiport Switch/23
  Hs and omega23/2(Hs n omega) -> Multiport Switch/24
  Hs and omega24/2(Hs n omega) -> Multiport Switch/25
  Count/1(switch signal) -> Multiport Switch/1
  Multiport Switch/1 -> Hs and omega/1
  Hs and omega1/1(Hs) -> Count/1(hs1)
  Hs and omega2/1(Hs) -> Count/2(hs2)
  Hs and omega3/1(Hs) -> Count/3(hs3)
  Hs and omega4/1(Hs) -> Count/4(hs4)
  Hs and omega5/1(Hs) -> Count/5(hs5)
  Hs and omega6/1(Hs) -> Count/6(hs6)
  Hs and omega7/1(Hs) -> Count/7(hs7)
  Hs and omega8/1(Hs) -> Count/8(hs8)
  Hs and omega9/1(Hs) -> Count/9(hs9)
  Hs and omega10/1(Hs) -> Count/10(hs10)
  Hs and omega11/1(Hs) -> Count/11(hs11)
  Hs and omega12/1(Hs) -> Count/12(hs12)
  Hs and omega13/1(Hs) -> Count/13(hs13)
  Hs and omega14/1(Hs) -> Count/14(hs14)
  Hs and omega15/1(Hs) -> Count/15(hs15)
  Hs and omega16/1(Hs) -> Count/16(hs16)
  Hs and omega17/1(Hs) -> Count/17(hs17)
  Hs and omega18/1(Hs) -> Count/18(hs18)
  Hs and omega19/1(Hs) -> Count/19(hs19)
  Hs and omega20/1(Hs) -> Count/20(hs20)
  Hs and omega21/1(Hs) -> Count/21(hs21)
  Hs and omega22/1(Hs) -> Count/22(hs22)
  Hs and omega23/1(Hs) -> Count/23(hs23)
  Hs and omega24/1(Hs) -> Terminator/1

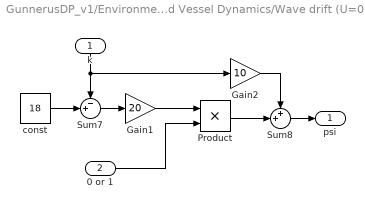
== system GunnerusDP_v1/Environment and Vessel Dynamics/Wave drift (U=0)/psi1 ==
  k : Inport
  0 or 1 : Inport  Port=2
  Gain1 : Gain  Gain=20
  Gain2 : Gain  Gain=10
  Product : Product  RndMeth=Zero
  Sum7 : Sum  Inputs=-+|
  Sum8 : Sum  Inputs=++|
  const : Constant  Value=18
  psi : Outport
  wires:
  const/1 -> Sum7/2
  Sum7/1 -> Gain1/1
  Gain1/1 -> Product/1
  Product/1 -> Sum8/2
  Gain2/1 -> Sum8/1
  k/1 -> Sum7/1, Gain2/1
  Sum8/1 -> psi/1
  0 or 1/1 -> Product/2

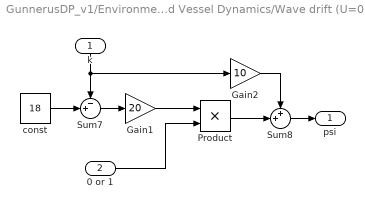
== system GunnerusDP_v1/Environment and Vessel Dynamics/Wave drift (U=0)/psi2 ==
  k : Inport
  0 or 1 : Inport  Port=2
  Gain1 : Gain  Gain=20
  Gain2 : Gain  Gain=10
  Product : Product  RndMeth=Zero
  Sum7 : Sum  Inputs=-+|
  Sum8 : Sum  Inputs=++|
  const : Constant  Value=18
  psi : Outport
  wires:
  const/1 -> Sum7/2
  Sum7/1 -> Gain1/1
  Gain1/1 -> Product/1
  Product/1 -> Sum8/2
  Gain2/1 -> Sum8/1
  k/1 -> Sum7/1, Gain2/1
  Sum8/1 -> psi/1
  0 or 1/1 -> Product/2

== system GunnerusDP_v1/Environment and Vessel Dynamics/6 DOF DP model (zero speed model with fluid memory)/Fluid memory effetcs/heave ==
  nu : Inport
  Selector : Selector  InputPortWidth=6  IndexOptions=Index vector (dialog)  Indices=[1]  OutputSizes=1
  Selector1 : Selector  InputPortWidth=6  IndexOptions=Index vector (dialog)  Indices=[3]  OutputSizes=1
  Selector2 : Selector  InputPortWidth=6  IndexOptions=Index vector (dialog)  Indices=[5]  OutputSizes=1
  u : Outport
  w : Outport  Port=2
  q : Outport  Port=3
  wires:
  Selector2/1 -> q/1
  Selector1/1 -> w/1
  Selector/1 -> u/1
  nu/1 -> Selector2/1, Selector1/1, Selector/1

== system GunnerusDP_v1/Environment and Vessel Dynamics/6 DOF DP model (zero speed model with fluid memory)/Fluid memory effetcs/pitch ==
  nu : Inport
  Selector : Selector  InputPortWidth=6  IndexOptions=Index vector (dialog)  Indices=[1]  OutputSizes=1
  Selector1 : Selector  InputPortWidth=6  IndexOptions=Index vector (dialog)  Indices=[3]  OutputSizes=1
  Selector2 : Selector  InputPortWidth=6  IndexOptions=Index vector (dialog)  Indices=[5]  OutputSizes=1
  u : Outport
  w : Outport  Port=2
  q : Outport  Port=3
  wires:
  Selector2/1 -> q/1
  Selector1/1 -> w/1
  Selector/1 -> u/1
  nu/1 -> Selector2/1, Selector1/1, Selector/1

== system GunnerusDP_v1/Environment and Vessel Dynamics/6 DOF DP model (zero speed model with fluid memory)/Fluid memory effetcs/roll ==
  nu : Inport
  Selector : Selector  InputPortWidth=6  IndexOptions=Index vector (dialog)  Indices=[2]  OutputSizes=1
  Selector1 : Selector  InputPortWidth=6  IndexOptions=Index vector (dialog)  Indices=[4]  OutputSizes=1
  Selector2 : Selector  InputPortWidth=6  IndexOptions=Index vector (dialog)  Indices=[6]  OutputSizes=1
  v : Outport
  p : Outport  Port=2
  r : Outport  Port=3
  wires:
  Selector2/1 -> r/1
  Selector1/1 -> p/1
  Selector/1 -> v/1
  nu/1 -> Selector2/1, Selector1/1, Selector/1

== system GunnerusDP_v1/Environment and Vessel Dynamics/6 DOF DP model (zero speed model with fluid memory)/Fluid memory effetcs/surge ==
  nu : Inport
  Selector : Selector  InputPortWidth=6  IndexOptions=Index vector (dialog)  Indices=[1]  OutputSizes=1
  Selector1 : Selector  InputPortWidth=6  IndexOptions=Index vector (dialog)  Indices=[3]  OutputSizes=1
  Selector2 : Selector  InputPortWidth=6  IndexOptions=Index vector (dialog)  Indices=[5]  OutputSizes=1
  u : Outport
  w : Outport  Port=2
  q : Outport  Port=3
  wires:
  Selector2/1 -> q/1
  Selector1/1 -> w/1
  Selector/1 -> u/1
  nu/1 -> Selector2/1, Selector1/1, Selector/1

== system GunnerusDP_v1/Environment and Vessel Dynamics/6 DOF DP model (zero speed model with fluid memory)/Fluid memory effetcs/sway ==
  nu : Inport
  Selector : Selector  InputPortWidth=6  IndexOptions=Index vector (dialog)  Indices=[2]  OutputSizes=1
  Selector1 : Selector  InputPortWidth=6  IndexOptions=Index vector (dialog)  Indices=[4]  OutputSizes=1
  Selector2 : Selector  InputPortWidth=6  IndexOptions=Index vector (dialog)  Indices=[6]  OutputSizes=1
  v : Outport
  p : Outport  Port=2
  r : Outport  Port=3
  wires:
  Selector2/1 -> r/1
  Selector1/1 -> p/1
  Selector/1 -> v/1
  nu/1 -> Selector2/1, Selector1/1, Selector/1

== system GunnerusDP_v1/Environment and Vessel Dynamics/6 DOF DP model (zero speed model with fluid memory)/Fluid memory effetcs/yaw ==
  nu : Inport
  Selector : Selector  InputPortWidth=6  IndexOptions=Index vector (dialog)  Indices=[2]  OutputSizes=1
  Selector1 : Selector  InputPortWidth=6  IndexOptions=Index vector (dialog)  Indices=[4]  OutputSizes=1
  Selector2 : Selector  InputPortWidth=6  IndexOptions=Index vector (dialog)  Indices=[6]  OutputSizes=1
  v : Outport
  p : Outport  Port=2
  r : Outport  Port=3
  wires:
  Selector2/1 -> r/1
  Selector1/1 -> p/1
  Selector/1 -> v/1
  nu/1 -> Selector2/1, Selector1/1, Selector/1

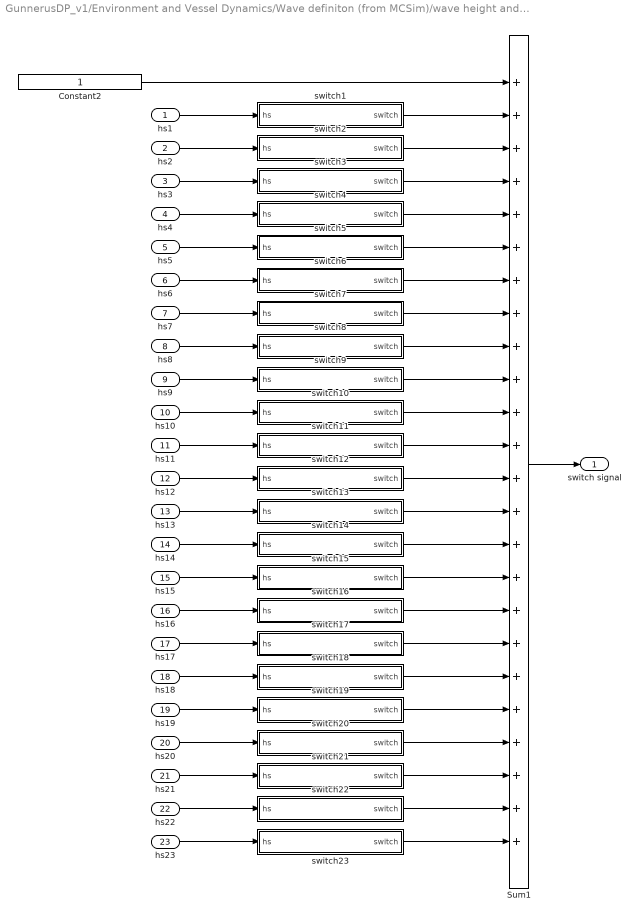
== system GunnerusDP_v1/Environment and Vessel Dynamics/Wave definiton (from MCSim)/wave height and wave frequency/Count ==
  hs1 : Inport
  hs2 : Inport  Port=2
  hs3 : Inport  Port=3
  hs4 : Inport  Port=4
  hs5 : Inport  Port=5
  hs6 : Inport  Port=6
  hs7 : Inport  Port=7
  hs8 : Inport  Port=8
  hs9 : Inport  Port=9
  hs10 : Inport  Port=10
  hs11 : Inport  Port=11
  hs12 : Inport  Port=12
  hs13 : Inport  Port=13
  hs14 : Inport  Port=14
  hs15 : Inport  Port=15
  hs16 : Inport  Port=16
  hs17 : Inport  Port=17
  hs18 : Inport  Port=18
  hs19 : Inport  Port=19
  hs20 : Inport  Port=20
  hs21 : Inport  Port=21
  hs22 : Inport  Port=22
  hs23 : Inport  Port=23
  Constant2 : Constant
  Sum1 : Sum  Inputs=++++++++++++++++++++++++  SaturateOnIntegerOverflow=on
  switch1 : Subsystem  mask{a=Par.Wave.hs(1), b=Par.Wave.hs(2)}
      mask prompts: a "Par.Wave.hs(i)=a"; b "Par.Wave.hs(i+1)=b"
  switch10 : Subsystem  mask{a=Par.Wave.hs(10), b=Par.Wave.hs(11)}
      mask prompts: a "Par.Wave.hs(i)=a"; b "Par.Wave.hs(i+1)=b"
  switch11 : Subsystem  mask{a=Par.Wave.hs(11), b=Par.Wave.hs(12)}
      mask prompts: a "Par.Wave.hs(i)=a"; b "Par.Wave.hs(i+1)=b"
  switch12 : Subsystem  mask{a=Par.Wave.hs(12), b=Par.Wave.hs(13)}
      mask prompts: a "Par.Wave.hs(i)=a"; b "Par.Wave.hs(i+1)=b"
  switch13 : Subsystem  mask{a=Par.Wave.hs(13), b=Par.Wave.hs(14)}
      mask prompts: a "Par.Wave.hs(i)=a"; b "Par.Wave.hs(i+1)=b"
  switch14 : Subsystem  mask{a=Par.Wave.hs(14), b=Par.Wave.hs(15)}
      mask prompts: a "Par.Wave.hs(i)=a"; b "Par.Wave.hs(i+1)=b"
  switch15 : Subsystem  mask{a=Par.Wave.hs(15), b=Par.Wave.hs(16)}
      mask prompts: a "Par.Wave.hs(i)=a"; b "Par.Wave.hs(i+1)=b"
  switch16 : Subsystem  mask{a=Par.Wave.hs(16), b=Par.Wave.hs(17)}
      mask prompts: a "Par.Wave.hs(i)=a"; b "Par.Wave.hs(i+1)=b"
  switch17 : Subsystem  mask{a=Par.Wave.hs(17), b=Par.Wave.hs(18)}
      mask prompts: a "Par.Wave.hs(i)=a"; b "Par.Wave.hs(i+1)=b"
  switch18 : Subsystem  mask{a=Par.Wave.hs(18), b=Par.Wave.hs(19)}
      mask prompts: a "Par.Wave.hs(i)=a"; b "Par.Wave.hs(i+1)=b"
  switch19 : Subsystem  mask{a=Par.Wave.hs(19), b=Par.Wave.hs(20)}
      mask prompts: a "Par.Wave.hs(i)=a"; b "Par.Wave.hs(i+1)=b"
  switch2 : Subsystem  mask{a=Par.Wave.hs(2), b=Par.Wave.hs(3)}
      mask prompts: a "Par.Wave.hs(i)=a"; b "Par.Wave.hs(i+1)=b"
  switch20 : Subsystem  mask{a=Par.Wave.hs(20), b=Par.Wave.hs(21)}
      mask prompts: a "Par.Wave.hs(i)=a"; b "Par.Wave.hs(i+1)=b"
  switch21 : Subsystem  mask{a=Par.Wave.hs(21), b=Par.Wave.hs(22)}
      mask prompts: a "Par.Wave.hs(i)=a"; b "Par.Wave.hs(i+1)=b"
  switch22 : Subsystem  mask{a=Par.Wave.hs(22), b=Par.Wave.hs(23)}
      mask prompts: a "Par.Wave.hs(i)=a"; b "Par.Wave.hs(i+1)=b"
  switch23 : Subsystem  mask{a=Par.Wave.hs(23), b=Par.Wave.hs(24)}
      mask prompts: a "Par.Wave.hs(i)=a"; b "Par.Wave.hs(i+1)=b"
  switch3 : Subsystem  mask{a=Par.Wave.hs(3), b=Par.Wave.hs(4)}
      mask prompts: a "Par.Wave.hs(i)=a"; b "Par.Wave.hs(i+1)=b"
  switch4 : Subsystem  mask{a=Par.Wave.hs(4), b=Par.Wave.hs(5)}
      mask prompts: a "Par.Wave.hs(i)=a"; b "Par.Wave.hs(i+1)=b"
  switch5 : Subsystem  mask{a=Par.Wave.hs(5), b=Par.Wave.hs(6)}
      mask prompts: a "Par.Wave.hs(i)=a"; b "Par.Wave.hs(i+1)=b"
  switch6 : Subsystem  mask{a=Par.Wave.hs(6), b=Par.Wave.hs(7)}
      mask prompts: a "Par.Wave.hs(i)=a"; b "Par.Wave.hs(i+1)=b"
  switch7 : Subsystem  mask{a=Par.Wave.hs(7), b=Par.Wave.hs(8)}
      mask prompts: a "Par.Wave.hs(i)=a"; b "Par.Wave.hs(i+1)=b"
  switch8 : Subsystem  mask{a=Par.Wave.hs(8), b=Par.Wave.hs(9)}
      mask prompts: a "Par.Wave.hs(i)=a"; b "Par.Wave.hs(i+1)=b"
  switch9 : Subsystem  mask{a=Par.Wave.hs(9), b=Par.Wave.hs(10)}
      mask prompts: a "Par.Wave.hs(i)=a"; b "Par.Wave.hs(i+1)=b"
  switch signal : Outport
  wires:
  hs1/1 -> switch1/1(hs)
  Sum1/1 -> switch signal/1
  Constant2/1 -> Sum1/1
  switch1/1(switch) -> Sum1/2
  hs2/1 -> switch2/1(hs)
  switch2/1(switch) -> Sum1/3
  hs3/1 -> switch3/1(hs)
  switch3/1(switch) -> Sum1/4
  hs4/1 -> switch4/1(hs)
  switch4/1(switch) -> Sum1/5
  hs5/1 -> switch5/1(hs)
  switch5/1(switch) -> Sum1/6
  hs6/1 -> switch6/1(hs)
  switch6/1(switch) -> Sum1/7
  hs7/1 -> switch7/1(hs)
  switch7/1(switch) -> Sum1/8
  hs8/1 -> switch8/1(hs)
  switch8/1(switch) -> Sum1/9
  hs9/1 -> switch9/1(hs)
  switch9/1(switch) -> Sum1/10
  hs10/1 -> switch10/1(hs)
  switch10/1(switch) -> Sum1/11
  hs11/1 -> switch11/1(hs)
  switch11/1(switch) -> Sum1/12
  hs12/1 -> switch12/1(hs)
  switch12/1(switch) -> Sum1/13
  hs13/1 -> switch13/1(hs)
  switch13/1(switch) -> Sum1/14
  hs14/1 -> switch14/1(hs)
  switch14/1(switch) -> Sum1/15
  hs15/1 -> switch15/1(hs)
  switch15/1(switch) -> Sum1/16
  hs16/1 -> switch16/1(hs)
  switch16/1(switch) -> Sum1/17
  hs17/1 -> switch17/1(hs)
  switch17/1(switch) -> Sum1/18
  hs18/1 -> switch18/1(hs)
  switch18/1(switch) -> Sum1/19
  hs19/1 -> switch19/1(hs)
  switch19/1(switch) -> Sum1/20
  hs20/1 -> switch20/1(hs)
  switch20/1(switch) -> Sum1/21
  hs21/1 -> switch21/1(hs)
  switch21/1(switch) -> Sum1/22
  hs22/1 -> switch22/1(hs)
  switch22/1(switch) -> Sum1/23
  hs23/1 -> switch23/1(hs)
  switch23/1(switch) -> Sum1/24

== system GunnerusDP_v1/Environment and Vessel Dynamics/Wave definiton (from MCSim)/wave height and wave frequency/Hs and omega1 ==
  t : Inport
  Mux : Mux  Inputs=2
  hs : Subsystem  mask{v1=Par.Wave.hs(1), v2=Par.Wave.hs(2), t1=Par.Wave.time_change(1), t2=Par.Wave.time_change(2)}
      mask prompts: v1 "value1"; v2 "value2"; t1 "time1"; t2 "time2"
      mask Display:
      | plot([0 1 4 5], [0 0 4 4])
      | port_label('output', 1, 'y')
      | port_label('input', 1, 'time')
  omega_p : Subsystem  mask{v1=Par.Wave.omega_peak(1), v2=Par.Wave.omega_peak(2), t1=Par.Wave.time_change(1), t2=Par.Wave.time_change(2)}
      mask prompts: v1 "value1"; v2 "value2"; t1 "time1"; t2 "time2"
      mask Display:
      | plot([0 1 4 5], [0 0 4 4])
      | port_label('output', 1, 'y')
      | port_label('input', 1, 'time')
  Hs : Outport
  Hs n omega : Outport  Port=2
  wires:
  t/1 -> omega_p/1(time), hs/1(time)
  hs/1(omega_peak) -> Hs/1, Mux/1
  Mux/1 -> Hs n omega/1
  omega_p/1(omega_peak) -> Mux/2

== system GunnerusDP_v1/Environment and Vessel Dynamics/Wave definiton (from MCSim)/wave height and wave frequency/Hs and omega10 ==
  t : Inport
  Mux : Mux  Inputs=2
  hs : Subsystem  mask{v1=Par.Wave.hs(10), v2=Par.Wave.hs(11), t1=Par.Wave.time_change(19), t2=Par.Wave.time_change(20)}
      mask prompts: v1 "value1"; v2 "value2"; t1 "time1"; t2 "time2"
      mask Display:
      | plot([0 1 4 5], [0 0 4 4])
      | port_label('output', 1, 'y')
      | port_label('input', 1, 'time')
  omega_p : Subsystem  mask{v1=Par.Wave.omega_peak(10), v2=Par.Wave.omega_peak(11), t1=Par.Wave.time_change(19), t2=Par.Wave.time_change(20)}
      mask prompts: v1 "value1"; v2 "value2"; t1 "time1"; t2 "time2"
      mask Display:
      | plot([0 1 4 5], [0 0 4 4])
      | port_label('output', 1, 'y')
      | port_label('input', 1, 'time')
  Hs : Outport
  Hs n omega : Outport  Port=2
  wires:
  omega_p/1(omega_peak) -> Mux/2
  Mux/1 -> Hs n omega/1
  hs/1(omega_peak) -> Mux/1, Hs/1
  t/1 -> hs/1(time), omega_p/1(time)

== system GunnerusDP_v1/Environment and Vessel Dynamics/Wave definiton (from MCSim)/wave height and wave frequency/Hs and omega11 ==
  t : Inport
  Mux : Mux  Inputs=2
  hs : Subsystem  mask{v1=Par.Wave.hs(11), v2=Par.Wave.hs(12), t1=Par.Wave.time_change(21), t2=Par.Wave.time_change(22)}
      mask prompts: v1 "value1"; v2 "value2"; t1 "time1"; t2 "time2"
      mask Display:
      | plot([0 1 4 5], [0 0 4 4])
      | port_label('output', 1, 'y')
      | port_label('input', 1, 'time')
  omega_p : Subsystem  mask{v1=Par.Wave.omega_peak(11), v2=Par.Wave.omega_peak(12), t1=Par.Wave.time_change(21), t2=Par.Wave.time_change(22)}
      mask prompts: v1 "value1"; v2 "value2"; t1 "time1"; t2 "time2"
      mask Display:
      | plot([0 1 4 5], [0 0 4 4])
      | port_label('output', 1, 'y')
      | port_label('input', 1, 'time')
  Hs : Outport
  Hs n omega : Outport  Port=2
  wires:
  t/1 -> omega_p/1(time), hs/1(time)
  hs/1(omega_peak) -> Hs/1, Mux/1
  Mux/1 -> Hs n omega/1
  omega_p/1(omega_peak) -> Mux/2

== system GunnerusDP_v1/Environment and Vessel Dynamics/Wave definiton (from MCSim)/wave height and wave frequency/Hs and omega12 ==
  t : Inport
  Mux : Mux  Inputs=2
  hs : Subsystem  mask{v1=Par.Wave.hs(12), v2=Par.Wave.hs(13), t1=Par.Wave.time_change(23), t2=Par.Wave.time_change(24)}
      mask prompts: v1 "value1"; v2 "value2"; t1 "time1"; t2 "time2"
      mask Display:
      | plot([0 1 4 5], [0 0 4 4])
      | port_label('output', 1, 'y')
      | port_label('input', 1, 'time')
  omega_p : Subsystem  mask{v1=Par.Wave.omega_peak(12), v2=Par.Wave.omega_peak(13), t1=Par.Wave.time_change(23), t2=Par.Wave.time_change(24)}
      mask prompts: v1 "value1"; v2 "value2"; t1 "time1"; t2 "time2"
      mask Display:
      | plot([0 1 4 5], [0 0 4 4])
      | port_label('output', 1, 'y')
      | port_label('input', 1, 'time')
  Hs : Outport
  Hs n omega : Outport  Port=2
  wires:
  omega_p/1(omega_peak) -> Mux/2
  Mux/1 -> Hs n omega/1
  hs/1(omega_peak) -> Mux/1, Hs/1
  t/1 -> hs/1(time), omega_p/1(time)

== system GunnerusDP_v1/Environment and Vessel Dynamics/Wave definiton (from MCSim)/wave height and wave frequency/Hs and omega13 ==
  t : Inport
  Mux : Mux  Inputs=2
  hs : Subsystem  mask{v1=Par.Wave.hs(13), v2=Par.Wave.hs(14), t1=Par.Wave.time_change(25), t2=Par.Wave.time_change(26)}
      mask prompts: v1 "value1"; v2 "value2"; t1 "time1"; t2 "time2"
      mask Display:
      | plot([0 1 4 5], [0 0 4 4])
      | port_label('output', 1, 'y')
      | port_label('input', 1, 'time')
  omega_p : Subsystem  mask{v1=Par.Wave.omega_peak(13), v2=Par.Wave.omega_peak(14), t1=Par.Wave.time_change(25), t2=Par.Wave.time_change(26)}
      mask prompts: v1 "value1"; v2 "value2"; t1 "time1"; t2 "time2"
      mask Display:
      | plot([0 1 4 5], [0 0 4 4])
      | port_label('output', 1, 'y')
      | port_label('input', 1, 'time')
  Hs : Outport
  Hs n omega : Outport  Port=2
  wires:
  t/1 -> omega_p/1(time), hs/1(time)
  hs/1(omega_peak) -> Hs/1, Mux/1
  Mux/1 -> Hs n omega/1
  omega_p/1(omega_peak) -> Mux/2

== system GunnerusDP_v1/Environment and Vessel Dynamics/Wave definiton (from MCSim)/wave height and wave frequency/Hs and omega14 ==
  t : Inport
  Mux : Mux  Inputs=2
  hs : Subsystem  mask{v1=Par.Wave.hs(14), v2=Par.Wave.hs(15), t1=Par.Wave.time_change(27), t2=Par.Wave.time_change(28)}
      mask prompts: v1 "value1"; v2 "value2"; t1 "time1"; t2 "time2"
      mask Display:
      | plot([0 1 4 5], [0 0 4 4])
      | port_label('output', 1, 'y')
      | port_label('input', 1, 'time')
  omega_p : Subsystem  mask{v1=Par.Wave.omega_peak(14), v2=Par.Wave.omega_peak(15), t1=Par.Wave.time_change(27), t2=Par.Wave.time_change(28)}
      mask prompts: v1 "value1"; v2 "value2"; t1 "time1"; t2 "time2"
      mask Display:
      | plot([0 1 4 5], [0 0 4 4])
      | port_label('output', 1, 'y')
      | port_label('input', 1, 'time')
  Hs : Outport
  Hs n omega : Outport  Port=2
  wires:
  omega_p/1(omega_peak) -> Mux/2
  Mux/1 -> Hs n omega/1
  hs/1(omega_peak) -> Mux/1, Hs/1
  t/1 -> hs/1(time), omega_p/1(time)

== system GunnerusDP_v1/Environment and Vessel Dynamics/Wave definiton (from MCSim)/wave height and wave frequency/Hs and omega15 ==
  t : Inport
  Mux : Mux  Inputs=2
  hs : Subsystem  mask{v1=Par.Wave.hs(15), v2=Par.Wave.hs(16), t1=Par.Wave.time_change(29), t2=Par.Wave.time_change(30)}
      mask prompts: v1 "value1"; v2 "value2"; t1 "time1"; t2 "time2"
      mask Display:
      | plot([0 1 4 5], [0 0 4 4])
      | port_label('output', 1, 'y')
      | port_label('input', 1, 'time')
  omega_p : Subsystem  mask{v1=Par.Wave.omega_peak(15), v2=Par.Wave.omega_peak(16), t1=Par.Wave.time_change(29), t2=Par.Wave.time_change(30)}
      mask prompts: v1 "value1"; v2 "value2"; t1 "time1"; t2 "time2"
      mask Display:
      | plot([0 1 4 5], [0 0 4 4])
      | port_label('output', 1, 'y')
      | port_label('input', 1, 'time')
  Hs : Outport
  Hs n omega : Outport  Port=2
  wires:
  t/1 -> omega_p/1(time), hs/1(time)
  hs/1(omega_peak) -> Hs/1, Mux/1
  Mux/1 -> Hs n omega/1
  omega_p/1(omega_peak) -> Mux/2

== system GunnerusDP_v1/Environment and Vessel Dynamics/Wave definiton (from MCSim)/wave height and wave frequency/Hs and omega16 ==
  t : Inport
  Mux : Mux  Inputs=2
  hs : Subsystem  mask{v1=Par.Wave.hs(16), v2=Par.Wave.hs(17), t1=Par.Wave.time_change(31), t2=Par.Wave.time_change(32)}
      mask prompts: v1 "value1"; v2 "value2"; t1 "time1"; t2 "time2"
      mask Display:
      | plot([0 1 4 5], [0 0 4 4])
      | port_label('output', 1, 'y')
      | port_label('input', 1, 'time')
  omega_p : Subsystem  mask{v1=Par.Wave.omega_peak(16), v2=Par.Wave.omega_peak(17), t1=Par.Wave.time_change(31), t2=Par.Wave.time_change(32)}
      mask prompts: v1 "value1"; v2 "value2"; t1 "time1"; t2 "time2"
      mask Display:
      | plot([0 1 4 5], [0 0 4 4])
      | port_label('output', 1, 'y')
      | port_label('input', 1, 'time')
  Hs : Outport
  Hs n omega : Outport  Port=2
  wires:
  t/1 -> omega_p/1(time), hs/1(time)
  hs/1(omega_peak) -> Hs/1, Mux/1
  Mux/1 -> Hs n omega/1
  omega_p/1(omega_peak) -> Mux/2
